simulink model "demo_lab6"  (R2023a)
settings: Solver=VariableStepAuto  StartTime=0.0  StopTime=300  RelTol=1e-3
settings Model: Creator=Dylan  LastModifiedBy=Dylan

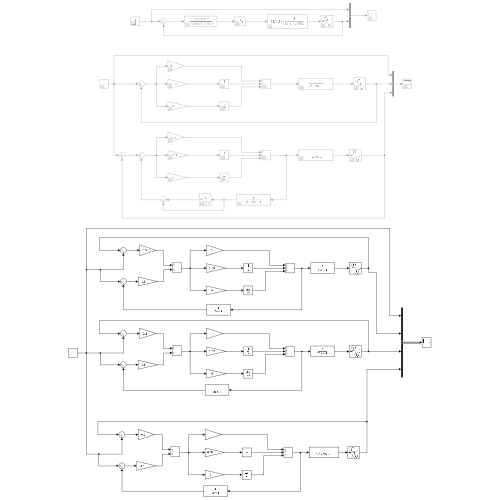
[thumbnail: Simulink's stored preview of the top-level diagram]
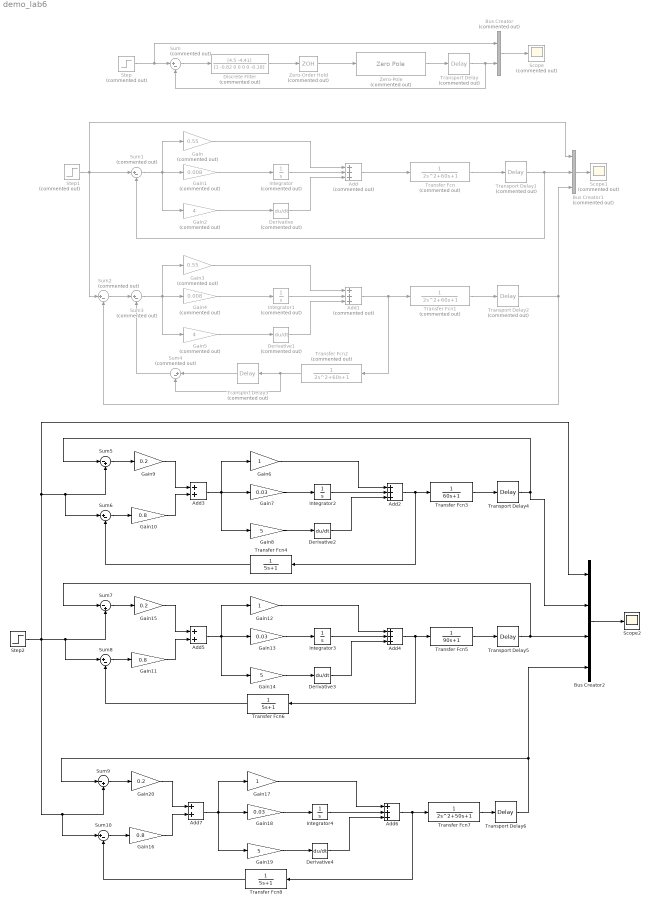
== system demo_lab6 ==
  Add : Sum  Commented=on  Inputs=+++
  Add1 : Sum  Commented=on  Inputs=+++
  Add2 : Sum  Inputs=+++
  Add3 : Sum
  Add4 : Sum  Inputs=+++
  Add5 : Sum
  Add6 : Sum  Inputs=+++
  Add7 : Sum
  Bus Creator : BusCreator  Commented=on  Inputs=2
  Bus Creator1 : BusCreator  Commented=on  Inputs=3
  Bus Creator2 : BusCreator  Inputs=4
  Derivative : Derivative  Commented=on
  Derivative1 : Derivative  Commented=on
  Derivative2 : Derivative
  Derivative3 : Derivative
  Derivative4 : Derivative
  Discrete Filter : DiscreteFilter  Commented=on  Numerator=[4.5 -4.41]  Denominator=[1 -0.82 0 0 0 0 -0.18]  SampleTime=2
  Gain : Gain  Commented=on  Gain=0.55
  Gain1 : Gain  Commented=on  Gain=0.008
  Gain10 : Gain  Gain=0.8
  Gain11 : Gain  Gain=0.8
  Gain12 : Gain
  Gain13 : Gain  Gain=0.03
  Gain14 : Gain  Gain=5
  Gain15 : Gain  Gain=0.2
  Gain16 : Gain  Gain=0.8
  Gain17 : Gain
  Gain18 : Gain  Gain=0.03
  Gain19 : Gain  Gain=5
  Gain2 : Gain  Commented=on  Gain=4
  Gain20 : Gain  Gain=0.2
  Gain3 : Gain  Commented=on  Gain=0.55
  Gain4 : Gain  Commented=on  Gain=0.008
  Gain5 : Gain  Commented=on  Gain=4
  Gain6 : Gain
  Gain7 : Gain  Gain=0.03
  Gain8 : Gain  Gain=5
  Gain9 : Gain  Gain=0.2
  Integrator : Integrator  Commented=on
  Integrator1 : Integrator  Commented=on
  Integrator2 : Integrator
  Integrator3 : Integrator
  Integrator4 : Integrator
  Scope : Scope  Commented=on
  Scope1 : Scope  Commented=on
  Scope2 : Scope
  Step : Step  Commented=on  Time=0  SampleTime=0
  Step1 : Step  Commented=on  Time=0  SampleTime=2
  Step2 : Step  Time=0  SampleTime=2
  Sum{,1..4} (5 alike) : Sum  Commented=on  Inputs=|+-
  Sum10 : Sum  Inputs=|+-
  Sum5 : Sum  Inputs=|-+
  Sum6 : Sum  Inputs=|+-
  Sum7 : Sum  Inputs=|-+
  Sum8 : Sum  Inputs=|+-
  Sum9 : Sum  Inputs=|-+
  Transfer Fcn : TransferFcn  Commented=on  Denominator=[2 60 1]
  Transfer Fcn1 : TransferFcn  Commented=on  Denominator=[2 60 1]
  Transfer Fcn2 : TransferFcn  Commented=on  Denominator=[2 60 1]
  Transfer Fcn3 : TransferFcn  Denominator=[60 1]
  Transfer Fcn4 : TransferFcn  Denominator=[5 1]
  Transfer Fcn5 : TransferFcn  Denominator=[90 1]
  Transfer Fcn6 : TransferFcn  Denominator=[5 1]
  Transfer Fcn7 : TransferFcn  Denominator=[2 50 1]
  Transfer Fcn8 : TransferFcn  Denominator=[5 1]
  Transport Delay : TransportDelay  Commented=on  DelayTime=10
  Transport Delay1 : TransportDelay  Commented=on  DelayTime=30
  Transport Delay2 : TransportDelay  Commented=on  DelayTime=30
  Transport Delay3 : TransportDelay  Commented=on  DelayTime=30
  Transport Delay4 : TransportDelay  DelayTime=30
  Transport Delay5 : TransportDelay  DelayTime=30
  Transport Delay6 : TransportDelay  DelayTime=30
  Zero-Order Hold : ZeroOrderHold  Commented=on  SampleTime=-1
  Zero-Pole : ZeroPole  Commented=on  Zeros=[]  Poles=[-1/100]  Gain=[1/50]
  wires:
  Step/1 -> Bus Creator/1, Sum/1
  Sum/1 -> Discrete Filter/1
  Discrete Filter/1 -> Zero-Order Hold/1
  Zero-Order Hold/1 -> Zero-Pole/1
  Zero-Pole/1 -> Transport Delay/1
  Transport Delay/1 -> Sum/2, Bus Creator/2
  Bus Creator/1 -> Scope/1
  Bus Creator1/1 -> Scope1/1
  Gain/1 -> Add/1
  Gain1/1 -> Integrator/1
  Integrator/1 -> Add/2
  Derivative/1 -> Add/3
  Gain2/1 -> Derivative/1
  Add/1 -> Transfer Fcn/1
  Transfer Fcn/1 -> Transport Delay1/1
  Sum1/1 -> Gain2/1, Gain1/1, Gain/1
  Transport Delay1/1 -> Bus Creator1/2, Sum1/2
  Step1/1 -> Sum1/1, Bus Creator1/1, Sum2/1
  Derivative1/1 -> Add1/3
  Integrator1/1 -> Add1/2
  Gain3/1 -> Add1/1
  Gain5/1 -> Derivative1/1
  Add1/1 -> Transfer Fcn2/1, Transfer Fcn1/1
  Gain4/1 -> Integrator1/1
  Sum3/1 -> Gain5/1, Gain4/1, Gain3/1
  Sum2/1 -> Sum3/1
  Transfer Fcn1/1 -> Transport Delay2/1
  Transport Delay2/1 -> Bus Creator1/3, Sum2/2
  Transfer Fcn2/1 -> Sum4/2, Transport Delay3/1
  Transport Delay3/1 -> Sum4/1
  Sum4/1 -> Sum3/2
  Derivative2/1 -> Add2/3
  Integrator2/1 -> Add2/2
  Gain6/1 -> Add2/1
  Gain8/1 -> Derivative2/1
  Add2/1 -> Transfer Fcn4/1, Transfer Fcn3/1
  Gain7/1 -> Integrator2/1
  Add3/1 -> Gain8/1, Gain7/1, Gain6/1
  Transfer Fcn3/1 -> Transport Delay4/1
  Gain9/1 -> Add3/1
  Gain10/1 -> Add3/2
  Sum5/1 -> Gain9/1
  Transport Delay4/1 -> Sum5/1, Bus Creator2/2
  Sum6/1 -> Gain10/1
  Transfer Fcn4/1 -> Sum6/2
  Sum8/1 -> Gain11/1
  Sum7/1 -> Gain15/1
  Transport Delay5/1 -> Bus Creator2/3, Sum7/1
  Gain11/1 -> Add5/2
  Gain15/1 -> Add5/1
  Transfer Fcn6/1 -> Sum8/2
  Integrator3/1 -> Add4/2
  Gain12/1 -> Add4/1
  Add5/1 -> Gain14/1, Gain13/1, Gain12/1
  Gain14/1 -> Derivative3/1
  Gain13/1 -> Integrator3/1
  Add4/1 -> Transfer Fcn6/1, Transfer Fcn5/1
  Derivative3/1 -> Add4/3
  Transfer Fcn5/1 -> Transport Delay5/1
  Transfer Fcn7/1 -> Transport Delay6/1
  Derivative4/1 -> Add6/3
  Add6/1 -> Transfer Fcn8/1, Transfer Fcn7/1
  Gain18/1 -> Integrator4/1
  Add7/1 -> Gain19/1, Gain18/1, Gain17/1
  Step2/1 -> Bus Creator2/1, Sum6/1, Sum5/2, Sum10/1, Sum9/2, Sum8/1, Sum7/2
  Gain17/1 -> Add6/1
  Gain16/1 -> Add7/2
  Integrator4/1 -> Add6/2
  Gain19/1 -> Derivative4/1
  Transport Delay6/1 -> Bus Creator2/4, Sum9/1
  Transfer Fcn8/1 -> Sum10/2
  Sum10/1 -> Gain16/1
  Sum9/1 -> Gain20/1
  Gain20/1 -> Add7/1
  Bus Creator2/1 -> Scope2/1
